simulink model "motor_20160122_164527"  (R2014a)
settings: Solver=ode45  StartTime=0.0  StopTime=10.0  RelTol=1e-3
undefined symbols (not defined in the file): ECU_MOTOR, MDL
settings Model: Creator=yoshi12  LastModifiedBy=yoshi12

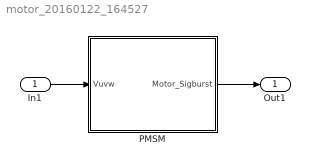
== system motor_20160122_164527 ==
  In1 : Inport  PortDimensions=3
  PMSM : Subsystem
  Out1 : Outport
  wires:
  In1/1 -> PMSM/1(Vuvw)
  PMSM/1(Motor_Sigburst) -> Out1/1

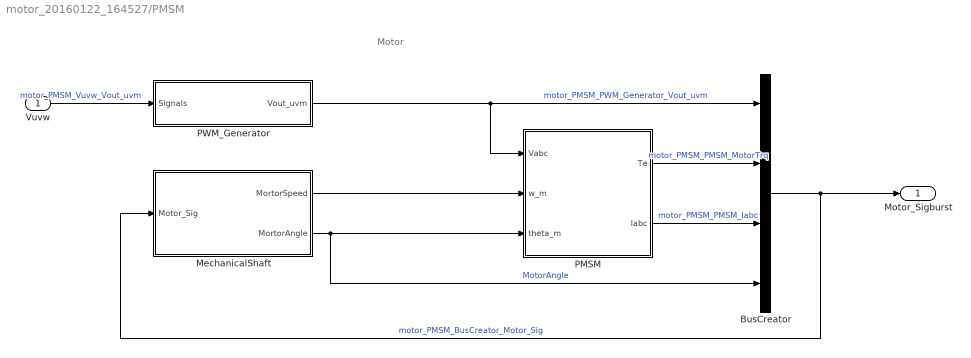
== system motor_20160122_164527/PMSM ==
  note: Motor
  Vuvw : Inport
  BusCreator : BusCreator
  MechanicalShaft : Subsystem  mask{Inertia=0.02, MaxRev=4e3, MinRev=0}
      mask prompts: Inertia "�ｽN�ｽ�ｽ�ｽ�ｽ�ｽN�ｽ�ｽ�ｽ�ｽ�ｽg�ｽ�ｽ�ｽN [kgm^2]"; MaxRev "�ｽﾅ托ｿｽ�ｽ]�ｽ�ｽ [rpm]"; MinRev "�ｽﾅ擾ｿｽ�ｽ�ｽ]�ｽ�ｽ [rpm]"
  PMSM : Subsystem  mask{R=MDL.MOTOR.R, p=MDL.MOTOR.p, Ld=MDL.MOTOR.Ld, Lq=MDL.MOTOR.Lq, Rnt=MDL.MOTOR.Rnt, JL=MDL.MOTOR.JL, KT=MDL.MOTOR.KT, ff=ECU_MOTOR.ff}
      mask prompts: R "�ｽ�ｽR(ohm)"; p "�ｽﾉ対撰ｿｽ"; Ld "d�ｽ�ｽ�ｽC�ｽ�ｽ�ｽ_�ｽN�ｽ^�ｽ�ｽ�ｽX�ｽiH�ｽj"; Lq "q�ｽ�ｽ�ｽC�ｽ�ｽ�ｽ_�ｽN�ｽ^�ｽ�ｽ�ｽX�ｽiH�ｽj"; Rnt "�ｽ�ｽ�ｽ�ｽ(V�ｽEs/rad)"; JL "�ｽ�ｽ�ｽ�ｽ�ｽ�ｽ�ｽ[�ｽ�ｽ�ｽ�ｽ�ｽg(kg�ｽEm�ｽO2)"; KT "�ｽg�ｽ�ｽ�ｽN�ｽ關( Nm/A)"
  PWM_Generator : Subsystem
  Motor_Sigburst : Outport  InitialOutput=0
  wires:
  BusCreator/1 -> Motor_Sigburst/1, MechanicalShaft/1(Motor_Sig)  "motor_PMSM_BusCreator_Motor_Sig"
  Vuvw/1 -> PWM_Generator/1(Signals)  "motor_PMSM_Vuvw_Vout_uvm"
  PMSM/2(Iabc) -> BusCreator/3  "motor_PMSM_PMSM_Iabc"
  PMSM/1(Te) -> BusCreator/2  "motor_PMSM_PMSM_MotorTrq"
  MechanicalShaft/2(MortorAngle) -> PMSM/3(theta_m), BusCreator/4  "MotorAngle"
  MechanicalShaft/1(MortorSpeed) -> PMSM/2(w_m)
  PWM_Generator/1(Vout_uvm) -> PMSM/1(Vabc), BusCreator/1  "motor_PMSM_PWM_Generator_Vout_uvm"

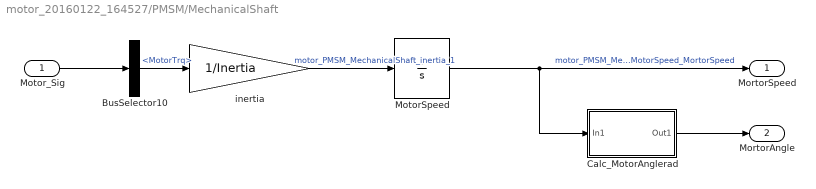
== system motor_20160122_164527/PMSM/MechanicalShaft ==
  Motor_Sig : Inport
  BusSelector10 : BusSelector  OutputSignals=MotorTrq
  Calc_MotorAnglerad : Subsystem
  MotorSpeed : Integrator  LimitOutput=on  UpperSaturationLimit=MaxRev*pi/30  LowerSaturationLimit=MinRev*pi/30
  inertia : Gain  Gain=1/Inertia  SaturateOnIntegerOverflow=on  OutDataTypeStr=Inherit: Same as input  ParamDataTypeStr=Inherit: Same as input
  MortorSpeed : Outport  InitialOutput=0
  MortorAngle : Outport  Port=2  InitialOutput=0
  wires:
  MotorSpeed/1 -> MortorSpeed/1, Calc_MotorAnglerad/1(In1)  "motor_PMSM_MechanicalShaft_MotorSpeed_MortorSpeed"
  inertia/1 -> MotorSpeed/1  "motor_PMSM_MechanicalShaft_inertia_1"
  Motor_Sig/1 -> BusSelector10/1
  BusSelector10/1 -> inertia/1  "<MotorTrq>"
  Calc_MotorAnglerad/1(Out1) -> MortorAngle/1

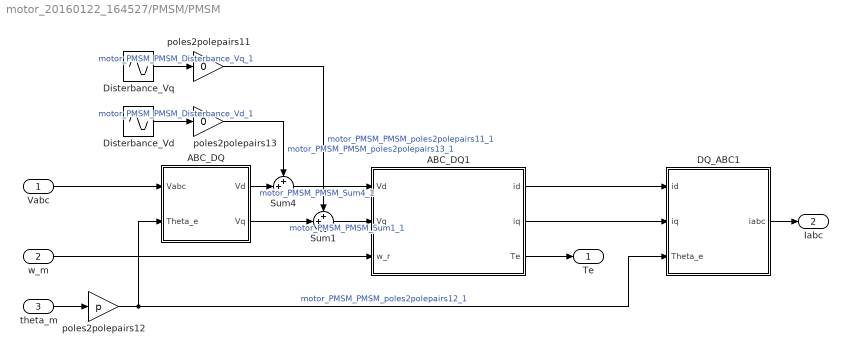
== system motor_20160122_164527/PMSM/PMSM ==
  Vabc : Inport
  w_m : Inport  Port=2
  theta_m : Inport  Port=3
  ABC_DQ : Subsystem
      mask Display: disp('abc-dq')
  ABC_DQ1 : Subsystem
      mask Display: disp('PMSM model')
  DQ_ABC1 : Subsystem
      mask Display: disp('dq-abc')
  Disterbance_Vd : Sin  Amplitude=5  Frequency=2*pi*ff  SampleTime=0
  Disterbance_Vq : Sin  Amplitude=5  Frequency=2*pi*ff  Phase=pi/2  SampleTime=0
  Sum1 : Sum  Inputs=++|
  Sum4 : Sum  Inputs=++|
  poles2polepairs11 : Gain  Gain=0
  poles2polepairs12 : Gain  Gain=p
  poles2polepairs13 : Gain  Gain=0
  Te : Outport
  Iabc : Outport  Port=2
  wires:
  poles2polepairs13/1 -> Sum4/1  "motor_PMSM_PMSM_poles2polepairs13_1"
  poles2polepairs11/1 -> Sum1/1  "motor_PMSM_PMSM_poles2polepairs11_1"
  poles2polepairs12/1 -> ABC_DQ/2(Theta_e), DQ_ABC1/3(Theta_e)  "motor_PMSM_PMSM_poles2polepairs12_1"
  Vabc/1 -> ABC_DQ/1(Vabc)
  DQ_ABC1/1(iabc) -> Iabc/1
  theta_m/1 -> poles2polepairs12/1
  w_m/1 -> ABC_DQ1/3(w_r)
  ABC_DQ1/2(iq) -> DQ_ABC1/2(iq)
  ABC_DQ1/1(id) -> DQ_ABC1/1(id)
  Disterbance_Vq/1 -> poles2polepairs11/1  "motor_PMSM_PMSM_Disterbance_Vq_1"
  Disterbance_Vd/1 -> poles2polepairs13/1  "motor_PMSM_PMSM_Disterbance_Vd_1"
  ABC_DQ/1(Vd) -> Sum4/2
  ABC_DQ/2(Vq) -> Sum1/2
  Sum4/1 -> ABC_DQ1/1(Vd)  "motor_PMSM_PMSM_Sum4_1"
  Sum1/1 -> ABC_DQ1/2(Vq)  "motor_PMSM_PMSM_Sum1_1"
  ABC_DQ1/3(Te) -> Te/1

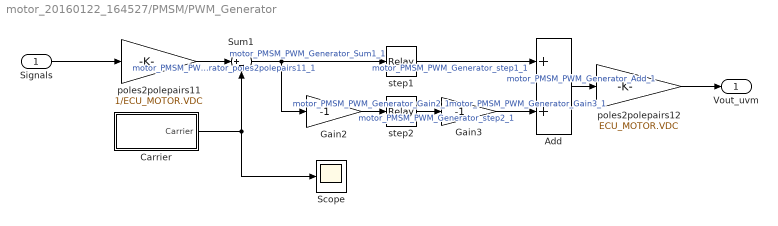
== system motor_20160122_164527/PMSM/PWM_Generator ==
  Signals : Inport
  Add : Sum
  Carrier : Subsystem  mask{Ts=1e-5, Freq=ECU_MOTOR.f_carrier}
      mask prompts: Ts "�ｽT�ｽ�ｽ�ｽv�ｽ�ｽ�ｽ�ｽ�ｽﾔ（Ts�ｽj"; Freq "�ｽ�ｽg�ｽ�ｽ(Freq)"
  Gain2 : Gain  Gain=-1  OutDataTypeStr=double
  Gain3 : Gain  Gain=-1  OutDataTypeStr=double
  Scope : Scope
  Sum1 : Sum  Inputs=|+-  SaturateOnIntegerOverflow=on  InputSameDT=on  OutDataTypeStr=Inherit: Same as first input
  poles2polepairs11 : Gain  Gain=1/ECU_MOTOR.VDC
  poles2polepairs12 : Gain  Gain=ECU_MOTOR.VDC
  step1 : Relay  OnSwitchValue=ECU_MOTOR.dvsw
  step2 : Relay  OnSwitchValue=ECU_MOTOR.dvsw
  Vout_uvm : Outport
  wires:
  Signals/1 -> poles2polepairs11/1
  Sum1/1 -> step1/1, Gain2/1  "motor_PMSM_PWM_Generator_Sum1_1"
  step1/1 -> Add/1  "motor_PMSM_PWM_Generator_step1_1"
  Gain2/1 -> step2/1  "motor_PMSM_PWM_Generator_Gain2_1"
  step2/1 -> Gain3/1  "motor_PMSM_PWM_Generator_step2_1"
  Gain3/1 -> Add/2  "motor_PMSM_PWM_Generator_Gain3_1"
  Add/1 -> poles2polepairs12/1  "motor_PMSM_PWM_Generator_Add_1"
  Carrier/1(Carrier) -> Sum1/2, Scope/1
  poles2polepairs11/1 -> Sum1/1  "motor_PMSM_PWM_Generator_poles2polepairs11_1"
  poles2polepairs12/1 -> Vout_uvm/1

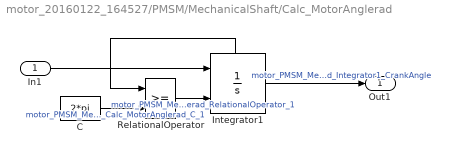
== system motor_20160122_164527/PMSM/MechanicalShaft/Calc_MotorAnglerad ==
  In1 : Inport
  C : Constant  Value=2*pi
  Integrator1 : Integrator  ExternalReset=rising  ShowStatePort=on
  RelationalOperator : RelationalOperator  OutDataTypeStr=boolean
  Out1 : Outport
  wires:
  Integrator1/1 -> Out1/1  "motor_PMSM_MechanicalShaft_Calc_MotorAnglerad_Integrator1_CrankAngle"
  In1/1 -> Integrator1/1
  Integrator1/State -> RelationalOperator/1
  C/1 -> RelationalOperator/2  "motor_PMSM_MechanicalShaft_Calc_MotorAnglerad_C_1"
  RelationalOperator/1 -> Integrator1/2  "motor_PMSM_MechanicalShaft_Calc_MotorAnglerad_RelationalOperator_1"

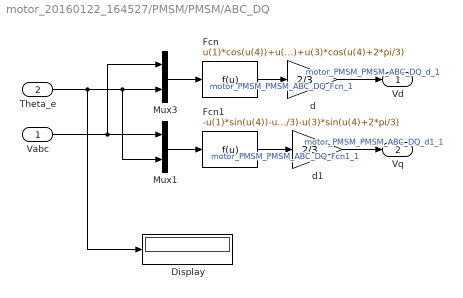
== system motor_20160122_164527/PMSM/PMSM/ABC_DQ ==
  Vabc : Inport
  Theta_e : Inport  Port=2
  Display : Display
  Fcn : Fcn  Expr=u(1)*cos(u(4))+u(2)*cos(u(4)-2*pi/3)+u(3)*cos(u(4)+2*pi/3)
  Fcn1 : Fcn  Expr=-u(1)*sin(u(4))-u(2)*sin(u(4)-2*pi/3)-u(3)*sin(u(4)+2*pi/3)
  Mux1 : Mux  Inputs=2
  Mux3 : Mux  Inputs=2
  d : Gain  Gain=2/3  OutDataTypeStr=Inherit: Same as input  ParamDataTypeStr=Inherit: Same as input
  d1 : Gain  Gain=2/3  OutDataTypeStr=Inherit: Same as input  ParamDataTypeStr=Inherit: Same as input
  Vd : Outport  InitialOutput=0
  Vq : Outport  Port=2  InitialOutput=0
  wires:
  d1/1 -> Vq/1  "motor_PMSM_PMSM_ABC_DQ_d1_1"
  d/1 -> Vd/1  "motor_PMSM_PMSM_ABC_DQ_d_1"
  Vabc/1 -> Mux3/1, Mux1/1
  Fcn1/1 -> d1/1  "motor_PMSM_PMSM_ABC_DQ_Fcn1_1"
  Mux1/1 -> Fcn1/1
  Fcn/1 -> d/1  "motor_PMSM_PMSM_ABC_DQ_Fcn_1"
  Mux3/1 -> Fcn/1
  Theta_e/1 -> Display/1, Mux1/2, Mux3/2

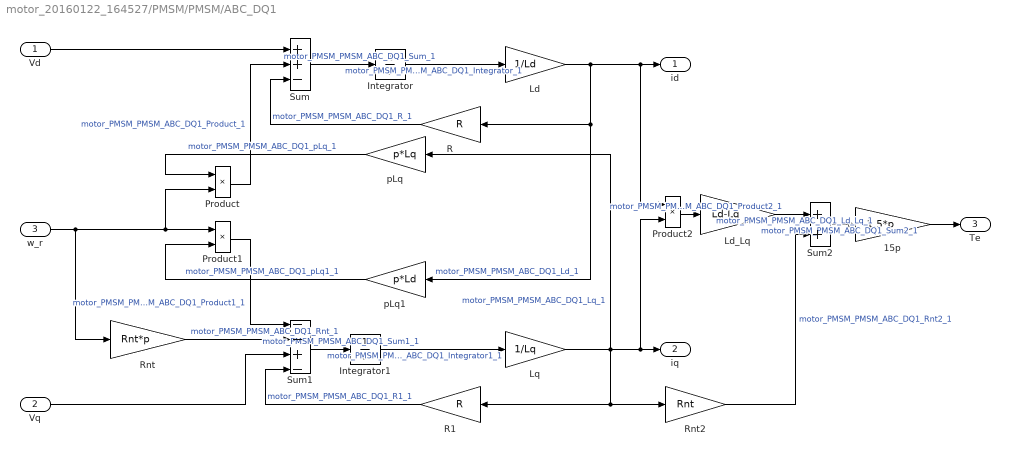
== system motor_20160122_164527/PMSM/PMSM/ABC_DQ1 ==
  Vd : Inport
  Vq : Inport  Port=2
  w_r : Inport  Port=3
  15p : Gain  Gain=1.5*p  SaturateOnIntegerOverflow=on  OutDataTypeStr=Inherit: Same as input  ParamDataTypeStr=Inherit: Same as input
  Integrator : Integrator
  Integrator1 : Integrator
  Ld : Gain  Gain=1/Ld  SaturateOnIntegerOverflow=on  OutDataTypeStr=Inherit: Same as input  ParamDataTypeStr=Inherit: Same as input
  Ld_Lq : Gain  Gain=Ld-Lq  SaturateOnIntegerOverflow=on  OutDataTypeStr=Inherit: Same as input  ParamDataTypeStr=Inherit: Same as input
  Lq : Gain  Gain=1/Lq  SaturateOnIntegerOverflow=on  OutDataTypeStr=Inherit: Same as input  ParamDataTypeStr=Inherit: Same as input
  Product : Product  SaturateOnIntegerOverflow=on  OutDataTypeStr=Inherit: Same as first input
  Product1 : Product  SaturateOnIntegerOverflow=on  OutDataTypeStr=Inherit: Same as first input
  Product2 : Product  SaturateOnIntegerOverflow=on  OutDataTypeStr=Inherit: Same as first input
  R : Gain  Gain=R  SaturateOnIntegerOverflow=on  OutDataTypeStr=Inherit: Same as input  ParamDataTypeStr=Inherit: Same as input
  R1 : Gain  Gain=R  SaturateOnIntegerOverflow=on  OutDataTypeStr=Inherit: Same as input  ParamDataTypeStr=Inherit: Same as input
  Rnt : Gain  Gain=Rnt*p  SaturateOnIntegerOverflow=on  OutDataTypeStr=Inherit: Same as input  ParamDataTypeStr=Inherit: Same as input
  Rnt2 : Gain  Gain=Rnt  SaturateOnIntegerOverflow=on  OutDataTypeStr=Inherit: Same as input  ParamDataTypeStr=Inherit: Same as input
  Sum : Sum  Inputs=++-  SaturateOnIntegerOverflow=on
  Sum1 : Sum  Inputs=--+-  SaturateOnIntegerOverflow=on
  Sum2 : Sum  SaturateOnIntegerOverflow=on
  pLq : Gain  Gain=p*Lq  SaturateOnIntegerOverflow=on  OutDataTypeStr=Inherit: Same as input  ParamDataTypeStr=Inherit: Same as input
  pLq1 : Gain  Gain=p*Ld  SaturateOnIntegerOverflow=on  OutDataTypeStr=Inherit: Same as input  ParamDataTypeStr=Inherit: Same as input
  id : Outport  InitialOutput=0
  iq : Outport  Port=2  InitialOutput=0
  Te : Outport  Port=3  InitialOutput=0
  wires:
  Vd/1 -> Sum/1
  Ld/1 -> R/1, pLq1/1, id/1, Product2/1  "motor_PMSM_PMSM_ABC_DQ1_Ld_1"
  R/1 -> Sum/3  "motor_PMSM_PMSM_ABC_DQ1_R_1"
  Sum1/1 -> Integrator1/1  "motor_PMSM_PMSM_ABC_DQ1_Sum1_1"
  Integrator1/1 -> Lq/1  "motor_PMSM_PMSM_ABC_DQ1_Integrator1_1"
  Lq/1 -> R1/1, Rnt2/1, iq/1, Product2/2, pLq/1  "motor_PMSM_PMSM_ABC_DQ1_Lq_1"
  Product/1 -> Sum/2  "motor_PMSM_PMSM_ABC_DQ1_Product_1"
  pLq/1 -> Product/1  "motor_PMSM_PMSM_ABC_DQ1_pLq_1"
  pLq1/1 -> Product1/2  "motor_PMSM_PMSM_ABC_DQ1_pLq1_1"
  Product1/1 -> Sum1/1  "motor_PMSM_PMSM_ABC_DQ1_Product1_1"
  w_r/1 -> Product/2, Product1/1, Rnt/1
  Vq/1 -> Sum1/3
  R1/1 -> Sum1/4  "motor_PMSM_PMSM_ABC_DQ1_R1_1"
  Rnt/1 -> Sum1/2  "motor_PMSM_PMSM_ABC_DQ1_Rnt_1"
  Sum2/1 -> 15p/1  "motor_PMSM_PMSM_ABC_DQ1_Sum2_1"
  15p/1 -> Te/1
  Rnt2/1 -> Sum2/2  "motor_PMSM_PMSM_ABC_DQ1_Rnt2_1"
  Product2/1 -> Ld_Lq/1  "motor_PMSM_PMSM_ABC_DQ1_Product2_1"
  Ld_Lq/1 -> Sum2/1  "motor_PMSM_PMSM_ABC_DQ1_Ld_Lq_1"
  Sum/1 -> Integrator/1  "motor_PMSM_PMSM_ABC_DQ1_Sum_1"
  Integrator/1 -> Ld/1  "motor_PMSM_PMSM_ABC_DQ1_Integrator_1"

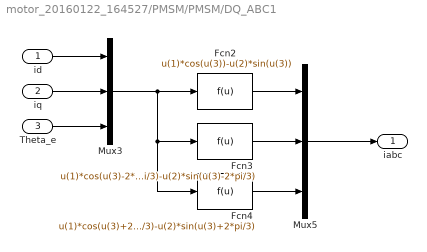
== system motor_20160122_164527/PMSM/PMSM/DQ_ABC1 ==
  id : Inport
  iq : Inport  Port=2
  Theta_e : Inport  Port=3
  Fcn2 : Fcn  Expr=u(1)*cos(u(3))-u(2)*sin(u(3))
  Fcn3 : Fcn  Expr=u(1)*cos(u(3)-2*pi/3)-u(2)*sin(u(3)-2*pi/3)
  Fcn4 : Fcn  Expr=u(1)*cos(u(3)+2*pi/3)-u(2)*sin(u(3)+2*pi/3)
  Mux3 : Mux  Inputs=3
  Mux5 : Mux  Inputs=3
  iabc : Outport  InitialOutput=0
  wires:
  Mux3/1 -> Fcn4/1, Fcn3/1, Fcn2/1
  Theta_e/1 -> Mux3/3
  iq/1 -> Mux3/2
  id/1 -> Mux3/1
  Fcn4/1 -> Mux5/3
  Fcn3/1 -> Mux5/2
  Mux5/1 -> iabc/1
  Fcn2/1 -> Mux5/1

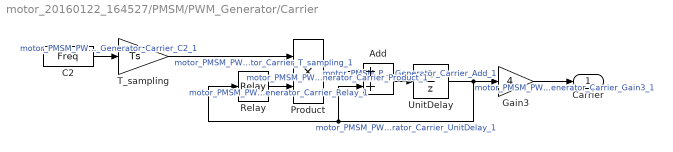
== system motor_20160122_164527/PMSM/PWM_Generator/Carrier ==
  Add : Sum
  C2 : Constant  Value=Freq
  Gain3 : Gain  Gain=4  OutDataTypeStr=double
  Product : Product  RndMeth=Zero
  Relay : Relay  OnSwitchValue=0.25  OffSwitchValue=-0.25  OnOutputValue=-1  OffOutputValue=1
  T_sampling : Gain  Gain=Ts
  UnitDelay : UnitDelay  SampleTime=-1
  Carrier : Outport
  wires:
  C2/1 -> T_sampling/1  "motor_PMSM_PWM_Generator_Carrier_C2_1"
  UnitDelay/1 -> Add/2, Relay/1, Gain3/1  "motor_PMSM_PWM_Generator_Carrier_UnitDelay_1"
  Add/1 -> UnitDelay/1  "motor_PMSM_PWM_Generator_Carrier_Add_1"
  T_sampling/1 -> Product/1  "motor_PMSM_PWM_Generator_Carrier_T_sampling_1"
  Relay/1 -> Product/2  "motor_PMSM_PWM_Generator_Carrier_Relay_1"
  Product/1 -> Add/1  "motor_PMSM_PWM_Generator_Carrier_Product_1"
  Gain3/1 -> Carrier/1  "motor_PMSM_PWM_Generator_Carrier_Gain3_1"
